simulink model "gm_sampleModel1659_sub"  (R2023a)
settings: Solver=VariableStepAuto  StartTime=0.0  StopTime=10.0  RelTol=1e-3
libraries: simulink x1
settings Model: Creator=user1  LastModifiedBy=user1
settings OptimizationCC: BlockReduction=off  ConditionallyExecuteInputs=off
settings DebuggingCC: InheritedTsInSrcMsg=none

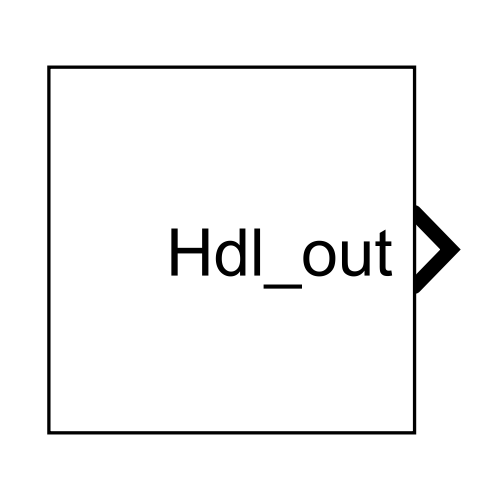
[thumbnail: Simulink's stored preview of the top-level diagram]
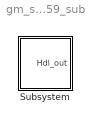
== system gm_sampleModel1659_sub ==
  Subsystem : Subsystem

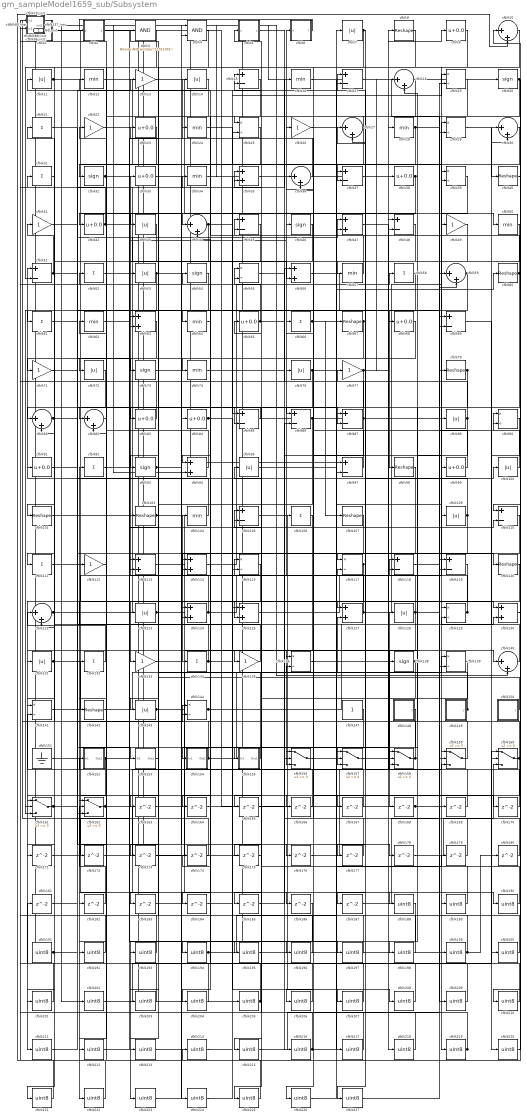
== system gm_sampleModel1659_sub/Subsystem ==
  cfblk1 : Subsystem  mask(Detect Fall Nonpositive){vinit=double(0), InputProcessing=Elements as channels (sample based), OutDataTypeStr=uint8}
      mask prompts: vinit "Simulink:masks:InitialCondition_MP"; InputProcessing "Simulink:masks:InputProcessing_MP"; OutDataTypeStr "Simulink:masks:OutputDataType_MP"
      mask help: Simulink:masks:DetectFallNonpositive_MD
      mask init:
      | InputProcessing = 'Elements as channels (sample based)';
      | OutDataTypeStr = 'uint8';
      | vinit = double(0);
      mask TypeOptions InputProcessing: Simulink:masks:ColumnsAsChannelsFrameBased | Simulink:masks:ElementsAsChannelsSampleBased
      mask TypeOptions OutDataTypeStr: Simulink:masks:uint8 | Simulink:masks:boolean
      mask Display: fprintf('U <= 0\n&  NOT\nU/z <= 0')
  cfblk{10,18,27,30,36,44,59,81..82,121,140} (11 alike) : Sum  Inputs=|++  OutDataTypeStr=uint8
  cfblk{7,11,14,43,53,72,76,89,95,100,109,123,128,131,143} (15 alike) : Abs  OutDataTypeStr=uint8  SaturateOnIntegerOverflow=off
  cfblk{8,40,60,67,79,98,101,103,107,120,142} (11 alike) : Reshape
  cfblk102_inst : Subsystem
  cfblk{12,16,24,28,34,50,57,62,64,74,104} (11 alike) : MinMax  OutDataTypeStr=uint8
  cfblk{15,17,37,45,48,51,69,85..87,97,105,110,118..119} (15 alike) : Sum  Inputs=+-  OutDataTypeStr=uint8
  cfblk{21,31,52,58,61,66,92,106,111,132,134} (11 alike) : Sum  Inputs=+  OutDataTypeStr=uint8
  cfblk108_inst : Subsystem
  cfblk{13,22,26,41,49,71,77,112,133,135} (10 alike) : Gain  OutDataTypeStr=uint8
  cfblk{35,47,56,63,94,113..114,124..125,127,130} (11 alike) : Sum  OutDataTypeStr=uint8
  cfblk{19,25,29,39,55,90,115,117,129,136,139,141,144} (13 alike) : Product  Inputs=*/  OutDataTypeStr=uint8  RndMeth=Zero  SaturateOnIntegerOverflow=on
  cfblk116_inst : Subsystem
  cfblk126_inst : Subsystem
  cfblk137_inst : Subsystem
  cfblk{20,32,46,54,73,93,138} (7 alike) : Signum
  cfblk147 : Constant  OutDataTypeStr=uint8  SampleTime=-1
  cfblk148 : Subsystem  mask(Counter Free-Running){NumBits=double(16), tsamp=double(-1)}
      mask prompts: NumBits "Simulink:masks:NumberOfBits_MP"; tsamp "Simulink:masks:SampleTime_MP"
      mask help: Simulink:masks:CounterFreeRunning_MD
  cfblk149 : Subsystem  mask(Counter Limited){uplimit=double(7), tsamp=double(-1)}
      mask prompts: uplimit "Simulink:masks:UpperLimit_MP"; tsamp "Simulink:masks:SampleTime_MP"
      mask help: Simulink:masks:CounterLimited_MD
      mask init:
      | nbits = double(8);
      | tsamp = double(-1);
      | uplimit = double(7);
  cfblk150 : Subsystem  mask(Counter Free-Running){NumBits=double(16), tsamp=double(-1)}
      mask prompts: NumBits "Simulink:masks:NumberOfBits_MP"; tsamp "Simulink:masks:SampleTime_MP"
      mask help: Simulink:masks:CounterFreeRunning_MD
  cfblk151 : Ground
  cfblk152 : Subsystem
  cfblk153 : Subsystem
  cfblk154 : Subsystem
  cfblk155 : Subsystem
  cfblk{156..162} (7 alike) : Switch  OutDataTypeStr=uint8  SaturateOnIntegerOverflow=off  InputSameDT=off
  cfblk{163..187} (25 alike) : Delay  SampleTime=1
  cfblk{188..227} (40 alike) : DataTypeConversion  OutDataTypeStr=uint8  SaturateOnIntegerOverflow=off  RndMeth=Floor
  cfblk2 : Subsystem  mask(Compare To Constant){relop=<=, const=double(3), OutDataTypeStr=uint8, ZeroCross=on}
      mask prompts: relop "Simulink:masks:Operator_MP"; const "Simulink:masks:ConstantValue_MP"; OutDataTypeStr "Simulink:masks:OutputDataType_MP"; ZeroCross "Simulink:masks:EnableZerocrossingDetection_MP"
      mask help: Simulink:masks:CompareToConstant_MD
      mask init:
      | OutDataTypeStr = 'uint8';
      | ZeroCross = 'on';
      | blkName = 'sampleModel1659_sub/Subsystem/cfblk2';
      | const = double(3);
      | const_str = '3.0';
      | const_val = double(3);
      | relop = '<=';
      | setValue = 'fixdt(0, 8)';
      | str = '<= 3';
      mask TypeOptions relop: == | ~= | < | <= | >= | >
      mask TypeOptions OutDataTypeStr: Simulink:masks:uint8 | Simulink:masks:boolean
      mask Callback ZeroCross: sl('zeroCrossEnable', gcbh);
      mask Display: disp(str)
  cfblk{9,23,33,38,42,65,68,83..84,91,99} (11 alike) : Bias  Bias=0.0  SaturateOnIntegerOverflow=off
  cfblk3 : simulink/Logic and Bit Operations/Bitwise Operator  logicop=AND  UseBitMask=on  BitMask=bin2dec('11011001')  BitMaskRealWorld=Stored Integer
      settings: LibrarySourceBlock=|
      | hdlsllib/Logic and Bit
      | Operations/Bitwise
      | Operator
  cfblk4 : Logic  AllPortsSameDT=off  OutDataTypeStr=boolean
  cfblk5 : Subsystem  mask(Compare To Constant){relop=<=, const=double(3), OutDataTypeStr=uint8, ZeroCross=on}
      mask prompts: relop "Simulink:masks:Operator_MP"; const "Simulink:masks:ConstantValue_MP"; OutDataTypeStr "Simulink:masks:OutputDataType_MP"; ZeroCross "Simulink:masks:EnableZerocrossingDetection_MP"
      mask help: Simulink:masks:CompareToConstant_MD
      mask init:
      | OutDataTypeStr = 'uint8';
      | ZeroCross = 'on';
      | blkName = 'sampleModel1659_sub/Subsystem/cfblk5';
      | const = double(3);
      | const_str = '3.0';
      | const_val = double(3);
      | relop = '<=';
      | setValue = 'fixdt(0, 8)';
      | str = '<= 3';
      mask TypeOptions relop: == | ~= | < | <= | >= | >
      mask TypeOptions OutDataTypeStr: Simulink:masks:uint8 | Simulink:masks:boolean
      mask Callback ZeroCross: sl('zeroCrossEnable', gcbh);
      mask Display: disp(str)
  cfblk6 : Subsystem  mask(Detect Rise Positive){vinit=double(0), InputProcessing=Elements as channels (sample based), OutDataTypeStr=uint8}
      mask prompts: vinit "Simulink:masks:InitialCondition_MP"; InputProcessing "Simulink:masks:InputProcessing_MP"; OutDataTypeStr "Simulink:masks:OutputDataType_MP"
      mask help: Simulink:masks:DetectRisePositive_MD
      mask init:
      | InputProcessing = 'Elements as channels (sample based)';
      | OutDataTypeStr = 'uint8';
      | vinit = double(0);
      mask TypeOptions InputProcessing: Simulink:masks:ColumnsAsChannelsFrameBased | Simulink:masks:ElementsAsChannelsSampleBased
      mask TypeOptions OutDataTypeStr: Simulink:masks:uint8 | Simulink:masks:boolean
      mask Display: fprintf('U > 0\n&  NOT\nU/z > 0')
  cfblk75_inst : Subsystem
  cfblk80_inst : Subsystem
  cfblk88_inst : Subsystem
  cfblk96_inst : Subsystem
  Hdl_out : Outport  OutDataTypeStr=uint8  SampleTime=1
  wires:
  cfblk1/1(Y) -> cfblk37/2, cfblk125/2
  cfblk10/1 -> cfblk219/1
  cfblk100/1 -> cfblk90/1
  cfblk101/1 -> cfblk33/1
  cfblk102_inst/1(out1) -> cfblk140/2
  cfblk103/1 -> cfblk190/1, cfblk157/3
  cfblk104/1 -> cfblk51/1
  cfblk105/1 -> cfblk208/1
  cfblk106/1 -> cfblk211/1
  cfblk107/1 -> cfblk134/1
  cfblk108_inst/1(out1) -> cfblk199/1
  cfblk109/1 -> cfblk27/2, cfblk215/1
  cfblk11/1 -> cfblk44/1, cfblk161/1
  cfblk110/1 -> cfblk159/1
  cfblk111/1 -> cfblk92/1
  cfblk112/1 -> cfblk22/1
  cfblk113/1 -> cfblk168/1
  cfblk114/1 -> cfblk58/1
  cfblk115/1 -> cfblk222/1
  cfblk116_inst/1(out1) -> cfblk38/1
  cfblk117/1 -> cfblk131/1, cfblk185/1, cfblk135/1
  cfblk118/1 -> cfblk169/1
  cfblk119/1 -> cfblk175/1
  cfblk12/1 -> cfblk217/1
  cfblk120/1 -> cfblk133/1
  cfblk121/1 -> cfblk47/1, cfblk129/1
  cfblk123/1 -> cfblk4/2, cfblk156/3
  cfblk124/1 -> cfblk117/2, cfblk104/1
  cfblk125/1 -> cfblk29/1
  cfblk126_inst/1(out1) -> cfblk94/2, cfblk89/1
  cfblk127/1 -> cfblk39/2, cfblk6/1(U)
  cfblk128/1 -> cfblk63/1, cfblk90/2, cfblk184/1, cfblk183/1
  cfblk129/1 -> cfblk76/1, cfblk118/1, cfblk13/1
  cfblk13/1 -> cfblk209/1
  cfblk130/1 -> cfblk214/1
  cfblk131/1 -> cfblk201/1, cfblk186/1
  cfblk132/1 -> cfblk121/1
  cfblk133/1 -> cfblk156/1
  cfblk134/1 -> cfblk91/1, cfblk207/1
  cfblk135/1 -> cfblk112/1
  cfblk136/1 -> cfblk48/2
  cfblk137_inst/1(out1) -> cfblk97/1
  cfblk138/1 -> cfblk227/1, cfblk196/1, cfblk187/1
  cfblk139/1 -> cfblk225/1
  cfblk14/1 -> cfblk182/1
  cfblk140/1 -> cfblk129/2
  cfblk141/1 -> cfblk8/1
  cfblk142/1 -> cfblk28/1
  cfblk143/1 -> cfblk69/1, cfblk127/2
  cfblk144/1 -> cfblk30/2, cfblk30/1
  cfblk147/1 -> cfblk192/1
  cfblk148/1(y) -> cfblk162/1
  cfblk149/1(y) -> cfblk36/1, cfblk103/1, cfblk77/1
  cfblk15/1 -> cfblk82/1
  cfblk150/1(y) -> cfblk53/1
  cfblk151/1 -> cfblk220/1
  cfblk152/1(Out1) -> cfblk113/1, cfblk171/1, cfblk52/1
  cfblk153/1(Out1) -> cfblk23/1
  cfblk154/1(Out1) -> cfblk59/1, cfblk31/1
  cfblk155/1(Out1) -> cfblk54/1
  cfblk156/1 -> cfblk67/1
  cfblk157/1 -> cfblk128/1
  cfblk158/1 -> cfblk17/1, cfblk116_inst/1(in1), cfblk66/1
  cfblk159/1 -> cfblk95/1
  cfblk16/1 -> cfblk157/1
  cfblk160/1 -> cfblk206/1, cfblk18/2
  cfblk161/1 -> cfblk125/1, cfblk100/1
  cfblk162/1 -> cfblk224/1, cfblk166/1
  cfblk163/1 -> cfblk29/2
  cfblk164/1 -> cfblk25/2
  cfblk165/1 -> cfblk86/2
  cfblk166/1 -> cfblk141/2
  cfblk167/1 -> cfblk15/1
  cfblk168/1 -> cfblk59/2, Hdl_out/1
  cfblk169/1 -> cfblk27/1
  cfblk17/1 -> cfblk119/1
  cfblk170/1 -> cfblk48/1
  cfblk171/1 -> cfblk63/2
  cfblk172/1 -> cfblk157/2
  cfblk173/1 -> cfblk158/2
  cfblk174/1 -> cfblk126_inst/2(in2)
  cfblk175/1 -> cfblk1/1(U)
  cfblk176/1 -> cfblk159/3
  cfblk177/1 -> cfblk156/2
  cfblk178/1 -> cfblk160/3
  cfblk179/1 -> cfblk136/2
  cfblk18/1 -> cfblk143/1
  cfblk180/1 -> cfblk159/2
  cfblk181/1 -> cfblk144/1
  cfblk182/1 -> cfblk162/2
  cfblk183/1 -> cfblk114/2
  cfblk184/1 -> cfblk130/2
  cfblk185/1 -> cfblk110/2
  cfblk186/1 -> cfblk223/1
  cfblk187/1 -> cfblk79/1
  cfblk188/1 -> cfblk193/1
  cfblk189/1 -> cfblk35/1
  cfblk19/1 -> cfblk213/1
  cfblk190/1 -> cfblk35/2
  cfblk191/1 -> cfblk47/2, cfblk34/1
  cfblk192/1 -> cfblk88_inst/1(in1)
  cfblk193/1 -> cfblk88_inst/2(in2)
  cfblk194/1 -> cfblk7/1, cfblk44/2
  cfblk195/1 -> cfblk45/1
  cfblk196/1 -> cfblk45/2
  cfblk197/1 -> cfblk3/1
  cfblk198/1 -> cfblk62/1
  cfblk199/1 -> cfblk102_inst/2(in2), cfblk180/1, cfblk12/1
  cfblk2/1(y) -> cfblk189/1
  cfblk20/1 -> cfblk94/1, cfblk210/1
  cfblk200/1 -> cfblk108_inst/1(in1)
  cfblk201/1 -> cfblk108_inst/2(in2)
  cfblk202/1 -> cfblk160/1
  cfblk203/1 -> cfblk75_inst/1(in1)
  cfblk204/1 -> cfblk75_inst/2(in2)
  cfblk205/1 -> cfblk96_inst/2(in2), cfblk181/1
  cfblk206/1 -> cfblk80_inst/1(in1)
  cfblk207/1 -> cfblk80_inst/2(in2)
  cfblk208/1 -> cfblk174/1
  cfblk209/1 -> cfblk105/1
  cfblk21/1 -> cfblk73/1
  cfblk210/1 -> cfblk105/2
  cfblk211/1 -> cfblk162/3
  cfblk212/1 -> cfblk106/1
  cfblk213/1 -> cfblk84/1
  cfblk214/1 -> cfblk19/1
  cfblk215/1 -> cfblk19/2
  cfblk216/1 -> cfblk65/1, cfblk179/1
  cfblk217/1 -> cfblk55/1
  cfblk218/1 -> cfblk55/2
  cfblk219/1 -> cfblk137_inst/1(in1), cfblk5/1(u)
  cfblk22/1 -> cfblk56/2
  cfblk220/1 -> cfblk10/1
  cfblk221/1 -> cfblk10/2
  cfblk222/1 -> cfblk126_inst/1(in1)
  cfblk223/1 -> cfblk115/1
  cfblk224/1 -> cfblk115/2
  cfblk225/1 -> cfblk152/1(In1)
  cfblk226/1 -> cfblk139/1
  cfblk227/1 -> cfblk139/2
  cfblk23/1 -> cfblk132/1
  cfblk24/1 -> cfblk39/1
  cfblk25/1 -> cfblk32/1
  cfblk26/1 -> cfblk97/2
  cfblk27/1 -> cfblk124/1, cfblk25/1
  cfblk28/1 -> cfblk87/2, cfblk130/1
  cfblk29/1 -> cfblk40/1
  cfblk3/1 -> cfblk42/1
  cfblk30/1 -> cfblk142/1
  cfblk31/1 -> cfblk61/1
  cfblk32/1 -> cfblk85/2, cfblk64/1
  cfblk33/1 -> cfblk178/1
  cfblk34/1 -> cfblk85/1
  cfblk35/1 -> cfblk188/1
  cfblk36/1 -> cfblk14/1
  cfblk37/1 -> cfblk9/1
  cfblk38/1 -> cfblk72/1, cfblk177/1
  cfblk39/1 -> cfblk49/1
  cfblk4/1 -> cfblk51/2
  cfblk40/1 -> cfblk110/1
  cfblk41/1 -> cfblk83/1
  cfblk42/1 -> cfblk124/2, cfblk102_inst/1(in1), cfblk16/1
  cfblk43/1 -> cfblk111/1
  cfblk44/1 -> cfblk82/2, cfblk69/2
  cfblk45/1 -> cfblk194/1
  cfblk46/1 -> cfblk203/1
  cfblk47/1 -> cfblk119/2
  cfblk48/1 -> cfblk93/1
  cfblk49/1 -> cfblk172/1
  cfblk5/1(y) -> cfblk50/1
  cfblk50/1 -> cfblk121/2
  cfblk51/1 -> cfblk113/2, cfblk41/1
  cfblk52/1 -> cfblk24/1
  cfblk53/1 -> cfblk161/3, cfblk155/1(In1)
  cfblk54/1 -> cfblk161/2
  cfblk55/1 -> cfblk216/1
  cfblk56/1 -> cfblk98/1
  cfblk57/1 -> cfblk11/1
  cfblk58/1 -> cfblk141/1
  cfblk59/1 -> cfblk164/1, cfblk144/2
  cfblk6/1(Y) -> cfblk2/1(u)
  cfblk60/1 -> cfblk198/1, cfblk26/1
  cfblk61/1 -> cfblk68/1
  cfblk62/1 -> cfblk197/1
  cfblk63/1 -> cfblk81/2
  cfblk64/1 -> cfblk114/1
  cfblk65/1 -> cfblk140/1, cfblk116_inst/2(in2)
  cfblk66/1 -> cfblk60/1, cfblk107/1
  cfblk67/1 -> cfblk127/1, cfblk71/1
  cfblk68/1 -> cfblk74/1
  cfblk69/1 -> cfblk200/1
  cfblk7/1 -> cfblk43/1, cfblk57/1
  cfblk71/1 -> cfblk15/2
  cfblk72/1 -> cfblk101/1
  cfblk73/1 -> cfblk167/1
  cfblk74/1 -> cfblk99/1
  cfblk75_inst/1(out1) -> cfblk202/1
  cfblk76/1 -> cfblk226/1, cfblk173/1, cfblk170/1
  cfblk77/1 -> cfblk218/1, cfblk195/1, cfblk18/1
  cfblk79/1 -> cfblk204/1, cfblk138/1, cfblk117/1
  cfblk8/1 -> cfblk86/1
  cfblk80_inst/1(out1) -> cfblk205/1
  cfblk81/1 -> cfblk176/1, cfblk153/1(In1)
  cfblk82/1 -> cfblk212/1
  cfblk83/1 -> cfblk21/1
  cfblk84/1 -> cfblk87/1, cfblk17/2, cfblk158/3
  cfblk85/1 -> cfblk81/1
  cfblk86/1 -> cfblk163/1, cfblk154/1(In1)
  cfblk87/1 -> cfblk56/1, cfblk136/1
  cfblk88_inst/1(out1) -> cfblk191/1
  cfblk89/1 -> cfblk96_inst/1(in1), cfblk4/1, cfblk158/1
  cfblk9/1 -> cfblk221/1
  cfblk90/1 -> cfblk160/2
  cfblk91/1 -> cfblk118/2
  cfblk92/1 -> cfblk46/1
  cfblk93/1 -> cfblk123/1, cfblk120/1
  cfblk94/1 -> cfblk137_inst/2(in2)
  cfblk95/1 -> cfblk109/1
  cfblk96_inst/1(out1) -> cfblk20/1
  cfblk97/1 -> cfblk36/2
  cfblk98/1 -> cfblk165/1
  cfblk99/1 -> cfblk37/1

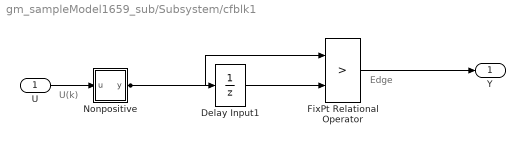
== system gm_sampleModel1659_sub/Subsystem/cfblk1 ==
  note: U(k)
  note: Edge
  U : Inport  OutDataTypeStr=uint8  SampleTime=1
  Delay Input1 : UnitDelay  Description=Store in Global RAM  DisableCoverage=on  InitialCondition=vinit  SampleTime=-1  HasFrameUpgradeWarning=on
  FixPt Relational Operator : RelationalOperator  Operator=>  OutDataTypeStr=fixdt(0, 8)  ZeroCross=off  InputSameDT=off
  Nonpositive : Subsystem  mask(Compare To Zero){relop=<=, OutDataTypeStr=boolean, ZeroCross=off}
      mask prompts: relop "Simulink:masks:Operator_MP"; OutDataTypeStr "Simulink:masks:OutputDataType_MP"; ZeroCross "Simulink:masks:EnableZerocrossingDetection_MP"
      mask help: Simulink:masks:CompareToZero_MD
      mask init:
      | OutDataTypeStr = 'boolean';
      | ZeroCross = 'off';
      | blkName = 'sampleModel1659_sub/Subsystem/cfblk1/Nonpositive';
      | relop = '<=';
      | setValue = 'boolean';
      mask TypeOptions relop: == | ~= | < | <= | >= | >
      mask TypeOptions OutDataTypeStr: Simulink:masks:uint8 | Simulink:masks:boolean
      mask Callback ZeroCross: sl('zeroCrossEnable', gcbh);
      mask Display: disp([relop,' 0'])
  Y : Outport  SampleTime=1
  wires:
  U/1 -> Nonpositive/1(u)
  Delay Input1/1 -> FixPt Relational Operator/2
  FixPt Relational Operator/1 -> Y/1
  Nonpositive/1(y) -> FixPt Relational Operator/1, Delay Input1/1

== system gm_sampleModel1659_sub/Subsystem/cfblk102_inst ==
  in1 : Inport  OutDataTypeStr=uint8  SampleTime=1
  in2 : Inport  Port=2  OutDataTypeStr=uint8  SampleTime=1
  mul_cfblk102_dotp_mulcomp : Product  Inputs=**  OutDataTypeStr=uint8  SampleTime=1
  out1 : Outport  OutDataTypeStr=uint8  SampleTime=1
  wires:
  in1/1 -> mul_cfblk102_dotp_mulcomp/1
  in2/1 -> mul_cfblk102_dotp_mulcomp/2
  mul_cfblk102_dotp_mulcomp/1 -> out1/1

== system gm_sampleModel1659_sub/Subsystem/cfblk108_inst ==
  in1 : Inport  OutDataTypeStr=uint8  SampleTime=1
  in2 : Inport  Port=2  OutDataTypeStr=uint8  SampleTime=1
  mul_cfblk108_dotp_mulcomp : Product  Inputs=**  OutDataTypeStr=uint8  SampleTime=1
  out1 : Outport  OutDataTypeStr=uint8  SampleTime=1
  wires:
  in1/1 -> mul_cfblk108_dotp_mulcomp/1
  in2/1 -> mul_cfblk108_dotp_mulcomp/2
  mul_cfblk108_dotp_mulcomp/1 -> out1/1

== system gm_sampleModel1659_sub/Subsystem/cfblk116_inst ==
  in1 : Inport  OutDataTypeStr=uint8  SampleTime=1
  in2 : Inport  Port=2  OutDataTypeStr=uint8  SampleTime=1
  mul_cfblk116_dotp_mulcomp : Product  Inputs=**  OutDataTypeStr=uint8  SampleTime=1
  out1 : Outport  OutDataTypeStr=uint8  SampleTime=1
  wires:
  in1/1 -> mul_cfblk116_dotp_mulcomp/1
  in2/1 -> mul_cfblk116_dotp_mulcomp/2
  mul_cfblk116_dotp_mulcomp/1 -> out1/1

== system gm_sampleModel1659_sub/Subsystem/cfblk126_inst ==
  in1 : Inport  OutDataTypeStr=uint8  SampleTime=1
  in2 : Inport  Port=2  OutDataTypeStr=uint8  SampleTime=1
  mul_cfblk126_dotp_mulcomp : Product  Inputs=**  OutDataTypeStr=uint8  SampleTime=1
  out1 : Outport  OutDataTypeStr=uint8  SampleTime=1
  wires:
  in1/1 -> mul_cfblk126_dotp_mulcomp/1
  in2/1 -> mul_cfblk126_dotp_mulcomp/2
  mul_cfblk126_dotp_mulcomp/1 -> out1/1

== system gm_sampleModel1659_sub/Subsystem/cfblk137_inst ==
  in1 : Inport  OutDataTypeStr=uint8  SampleTime=1
  in2 : Inport  Port=2  OutDataTypeStr=uint8  SampleTime=1
  mul_cfblk137_dotp_mulcomp : Product  Inputs=**  OutDataTypeStr=uint8  SampleTime=1
  out1 : Outport  OutDataTypeStr=uint8  SampleTime=1
  wires:
  in1/1 -> mul_cfblk137_dotp_mulcomp/1
  in2/1 -> mul_cfblk137_dotp_mulcomp/2
  mul_cfblk137_dotp_mulcomp/1 -> out1/1

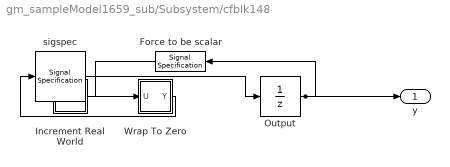
== system gm_sampleModel1659_sub/Subsystem/cfblk148 ==
  Force to be scalar : SignalSpecification  DisableCoverage=on  Dimensions=1
  Increment Real World : Subsystem  mask(Real World Value Increment){}
      mask help: Simulink:masks:RealWorldValueIncrement_MD
      mask Display: disp('V++')
  Output : UnitDelay  InitialCondition=0.0  SampleTime=tsamp  HasFrameUpgradeWarning=on
  Wrap To Zero : Subsystem  mask(Wrap To Zero){Threshold=double(65535)}
      mask prompts: Threshold "Simulink:masks:Threshold_MP"
      mask help: Simulink:masks:WrapToZero_MD
  sigspec : SignalSpecification  OutDataTypeStr=uint16  Dimensions=1
  y : Outport  SampleTime=1
  wires:
  Force to be scalar/1 -> Increment Real World/1(u)
  Increment Real World/1(y) -> Wrap To Zero/1(U)
  Output/1 -> Force to be scalar/1, y/1
  Wrap To Zero/1(Y) -> sigspec/1
  sigspec/1 -> Output/1

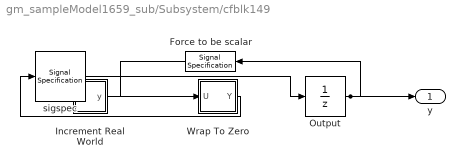
== system gm_sampleModel1659_sub/Subsystem/cfblk149 ==
  Force to be scalar : SignalSpecification  DisableCoverage=on  Dimensions=1
  Increment Real World : Subsystem  mask(Real World Value Increment){}
      mask help: Simulink:masks:RealWorldValueIncrement_MD
      mask Display: disp('V++')
  Output : UnitDelay  InitialCondition=0.0  SampleTime=tsamp  HasFrameUpgradeWarning=on
  Wrap To Zero : Subsystem  mask(Wrap To Zero){Threshold=double(7)}
      mask prompts: Threshold "Simulink:masks:Threshold_MP"
      mask help: Simulink:masks:WrapToZero_MD
  sigspec : SignalSpecification  OutDataTypeStr=uint8  Dimensions=1
  y : Outport  SampleTime=1
  wires:
  Force to be scalar/1 -> Increment Real World/1(u)
  Increment Real World/1(y) -> Wrap To Zero/1(U)
  Output/1 -> Force to be scalar/1, y/1
  Wrap To Zero/1(Y) -> sigspec/1
  sigspec/1 -> Output/1

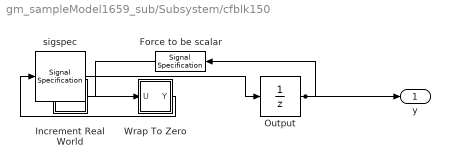
== system gm_sampleModel1659_sub/Subsystem/cfblk150 ==
  Force to be scalar : SignalSpecification  DisableCoverage=on  Dimensions=1
  Increment Real World : Subsystem  mask(Real World Value Increment){}
      mask help: Simulink:masks:RealWorldValueIncrement_MD
      mask Display: disp('V++')
  Output : UnitDelay  InitialCondition=0.0  SampleTime=tsamp  HasFrameUpgradeWarning=on
  Wrap To Zero : Subsystem  mask(Wrap To Zero){Threshold=double(65535)}
      mask prompts: Threshold "Simulink:masks:Threshold_MP"
      mask help: Simulink:masks:WrapToZero_MD
  sigspec : SignalSpecification  OutDataTypeStr=uint16  Dimensions=1
  y : Outport  SampleTime=1
  wires:
  Force to be scalar/1 -> Increment Real World/1(u)
  Increment Real World/1(y) -> Wrap To Zero/1(U)
  Output/1 -> Force to be scalar/1, y/1
  Wrap To Zero/1(Y) -> sigspec/1
  sigspec/1 -> Output/1

== system gm_sampleModel1659_sub/Subsystem/cfblk152 ==
  In1 : Inport  OutDataTypeStr=uint8  PortDimensions=1  SampleTime=1
  Out1 : Outport  SampleTime=1
  wires:
  In1/1 -> Out1/1

== system gm_sampleModel1659_sub/Subsystem/cfblk153 ==
  In1 : Inport  OutDataTypeStr=uint8  PortDimensions=1  SampleTime=1
  Out1 : Outport  SampleTime=1
  wires:
  In1/1 -> Out1/1

== system gm_sampleModel1659_sub/Subsystem/cfblk154 ==
  In1 : Inport  OutDataTypeStr=uint8  PortDimensions=1  SampleTime=1
  Out1 : Outport  SampleTime=1
  wires:
  In1/1 -> Out1/1

== system gm_sampleModel1659_sub/Subsystem/cfblk155 ==
  In1 : Inport  OutDataTypeStr=uint8  PortDimensions=1  SampleTime=1
  Out1 : Outport  SampleTime=1
  wires:
  In1/1 -> Out1/1

== system gm_sampleModel1659_sub/Subsystem/cfblk2 ==
  u : Inport  OutDataTypeStr=uint8  SampleTime=1
  Compare : RelationalOperator  Operator=<=  OutDataTypeStr=fixdt(0, 8)
  Constant : Constant  DisableCoverage=on  Value=const  OutDataTypeStr=Inherit: Inherit via back propagation  SampleTime=-1
  y : Outport  SampleTime=1
  wires:
  u/1 -> Compare/1
  Compare/1 -> y/1
  Constant/1 -> Compare/2

== system gm_sampleModel1659_sub/Subsystem/cfblk5 ==
  u : Inport  OutDataTypeStr=uint8  SampleTime=1
  Compare : RelationalOperator  Operator=<=  OutDataTypeStr=fixdt(0, 8)
  Constant : Constant  DisableCoverage=on  Value=const  OutDataTypeStr=Inherit: Inherit via back propagation  SampleTime=-1
  y : Outport  SampleTime=1
  wires:
  u/1 -> Compare/1
  Compare/1 -> y/1
  Constant/1 -> Compare/2

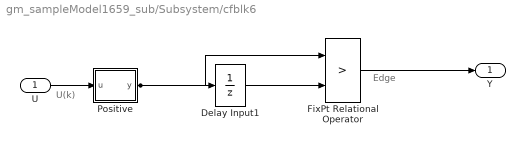
== system gm_sampleModel1659_sub/Subsystem/cfblk6 ==
  note: U(k)
  note: Edge
  U : Inport  OutDataTypeStr=uint8  SampleTime=1
  Delay Input1 : UnitDelay  Description=Store in Global RAM  DisableCoverage=on  InitialCondition=vinit  SampleTime=-1  HasFrameUpgradeWarning=on
  FixPt Relational Operator : RelationalOperator  Operator=>  OutDataTypeStr=fixdt(0, 8)  ZeroCross=off  InputSameDT=off
  Positive : Subsystem  mask(Compare To Zero){relop=>, OutDataTypeStr=boolean, ZeroCross=off}
      mask prompts: relop "Simulink:masks:Operator_MP"; OutDataTypeStr "Simulink:masks:OutputDataType_MP"; ZeroCross "Simulink:masks:EnableZerocrossingDetection_MP"
      mask help: Simulink:masks:CompareToZero_MD
      mask init:
      | OutDataTypeStr = 'boolean';
      | ZeroCross = 'off';
      | blkName = 'sampleModel1659_sub/Subsystem/cfblk6/Positive';
      | relop = '>';
      | setValue = 'boolean';
      mask TypeOptions relop: == | ~= | < | <= | >= | >
      mask TypeOptions OutDataTypeStr: Simulink:masks:uint8 | Simulink:masks:boolean
      mask Callback ZeroCross: sl('zeroCrossEnable', gcbh);
      mask Display: disp([relop,' 0'])
  Y : Outport  SampleTime=1
  wires:
  U/1 -> Positive/1(u)
  Delay Input1/1 -> FixPt Relational Operator/2
  FixPt Relational Operator/1 -> Y/1
  Positive/1(y) -> FixPt Relational Operator/1, Delay Input1/1

== system gm_sampleModel1659_sub/Subsystem/cfblk75_inst ==
  in1 : Inport  OutDataTypeStr=uint8  SampleTime=1
  in2 : Inport  Port=2  OutDataTypeStr=uint8  SampleTime=1
  mul_cfblk75_dotp_mulcomp : Product  Inputs=**  OutDataTypeStr=uint8  SampleTime=1
  out1 : Outport  OutDataTypeStr=uint8  SampleTime=1
  wires:
  in1/1 -> mul_cfblk75_dotp_mulcomp/1
  in2/1 -> mul_cfblk75_dotp_mulcomp/2
  mul_cfblk75_dotp_mulcomp/1 -> out1/1

== system gm_sampleModel1659_sub/Subsystem/cfblk80_inst ==
  in1 : Inport  OutDataTypeStr=uint8  SampleTime=1
  in2 : Inport  Port=2  OutDataTypeStr=uint8  SampleTime=1
  mul_cfblk80_dotp_mulcomp : Product  Inputs=**  OutDataTypeStr=uint8  SampleTime=1
  out1 : Outport  OutDataTypeStr=uint8  SampleTime=1
  wires:
  in1/1 -> mul_cfblk80_dotp_mulcomp/1
  in2/1 -> mul_cfblk80_dotp_mulcomp/2
  mul_cfblk80_dotp_mulcomp/1 -> out1/1

== system gm_sampleModel1659_sub/Subsystem/cfblk88_inst ==
  in1 : Inport  OutDataTypeStr=uint8  SampleTime=1
  in2 : Inport  Port=2  OutDataTypeStr=uint8  SampleTime=1
  mul_cfblk88_dotp_mulcomp : Product  Inputs=**  OutDataTypeStr=uint8  SampleTime=1
  out1 : Outport  OutDataTypeStr=uint8  SampleTime=1
  wires:
  in1/1 -> mul_cfblk88_dotp_mulcomp/1
  in2/1 -> mul_cfblk88_dotp_mulcomp/2
  mul_cfblk88_dotp_mulcomp/1 -> out1/1

== system gm_sampleModel1659_sub/Subsystem/cfblk96_inst ==
  in1 : Inport  OutDataTypeStr=uint8  SampleTime=1
  in2 : Inport  Port=2  OutDataTypeStr=uint8  SampleTime=1
  mul_cfblk96_dotp_mulcomp : Product  Inputs=**  OutDataTypeStr=uint8  SampleTime=1
  out1 : Outport  OutDataTypeStr=uint8  SampleTime=1
  wires:
  in1/1 -> mul_cfblk96_dotp_mulcomp/1
  in2/1 -> mul_cfblk96_dotp_mulcomp/2
  mul_cfblk96_dotp_mulcomp/1 -> out1/1

== system gm_sampleModel1659_sub/Subsystem/cfblk1/Nonpositive ==
  u : Inport  OutDataTypeStr=uint8  SampleTime=1
  Compare : RelationalOperator  Operator=<=  OutDataTypeStr=boolean  ZeroCross=off
  Constant : Constant  DisableCoverage=on  Value=0  OutDataTypeStr=Inherit: Inherit via back propagation  SampleTime=-1  PreserveConstantTs=on
  y : Outport  SampleTime=1
  wires:
  u/1 -> Compare/1
  Compare/1 -> y/1
  Constant/1 -> Compare/2

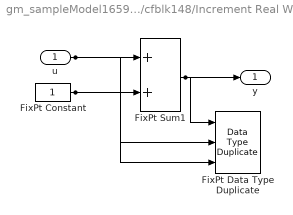
== system gm_sampleModel1659_sub/Subsystem/cfblk148/Increment Real World ==
  u : Inport  OutDataTypeStr=uint16  SampleTime=1
  FixPt Constant : Constant  DisableCoverage=on  OutDataTypeStr=Inherit: Inherit via back propagation  SampleTime=-1
  FixPt Data Type Duplicate : DataTypeDuplicate  DisableCoverage=on  NumInputPorts=3
  FixPt Sum1 : Sum  InputSameDT=on  OutDataTypeStr=Inherit: Inherit via back propagation  LockScale=on
  y : Outport  SampleTime=1
  wires:
  u/1 -> FixPt Sum1/1, FixPt Data Type Duplicate/2
  FixPt Constant/1 -> FixPt Sum1/2, FixPt Data Type Duplicate/3
  FixPt Sum1/1 -> FixPt Data Type Duplicate/1, y/1

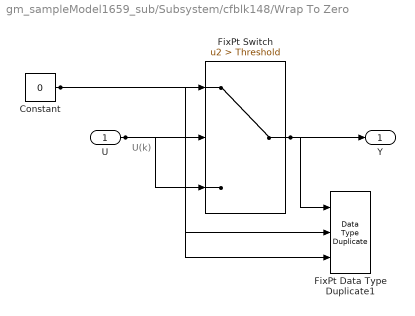
== system gm_sampleModel1659_sub/Subsystem/cfblk148/Wrap To Zero ==
  note: U(k)
  U : Inport  OutDataTypeStr=uint16  SampleTime=1
  Constant : Constant  DisableCoverage=on  Value=0  OutDataTypeStr=Inherit: Inherit via back propagation  SampleTime=-1
  FixPt Data Type Duplicate1 : DataTypeDuplicate  DisableCoverage=on  NumInputPorts=3
  FixPt Switch : Switch  Criteria=u2 > Threshold  Threshold=Threshold  OutDataTypeStr=Inherit: Inherit via back propagation  ZeroCross=off  SaturateOnIntegerOverflow=off  InputSameDT=off
  Y : Outport  SampleTime=1
  wires:
  U/1 -> FixPt Switch/3, FixPt Switch/2, FixPt Data Type Duplicate1/2
  Constant/1 -> FixPt Switch/1, FixPt Data Type Duplicate1/3
  FixPt Switch/1 -> FixPt Data Type Duplicate1/1, Y/1

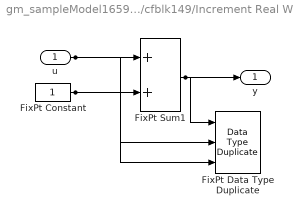
== system gm_sampleModel1659_sub/Subsystem/cfblk149/Increment Real World ==
  u : Inport  OutDataTypeStr=uint8  SampleTime=1
  FixPt Constant : Constant  DisableCoverage=on  OutDataTypeStr=Inherit: Inherit via back propagation  SampleTime=-1
  FixPt Data Type Duplicate : DataTypeDuplicate  DisableCoverage=on  NumInputPorts=3
  FixPt Sum1 : Sum  InputSameDT=on  OutDataTypeStr=Inherit: Inherit via back propagation  LockScale=on
  y : Outport  SampleTime=1
  wires:
  u/1 -> FixPt Sum1/1, FixPt Data Type Duplicate/2
  FixPt Constant/1 -> FixPt Sum1/2, FixPt Data Type Duplicate/3
  FixPt Sum1/1 -> FixPt Data Type Duplicate/1, y/1

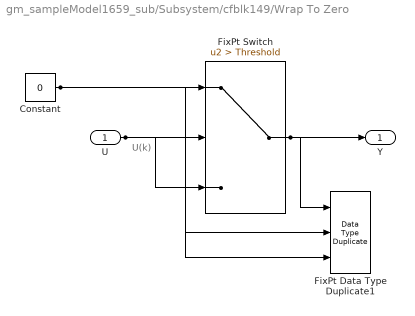
== system gm_sampleModel1659_sub/Subsystem/cfblk149/Wrap To Zero ==
  note: U(k)
  U : Inport  OutDataTypeStr=uint8  SampleTime=1
  Constant : Constant  DisableCoverage=on  Value=0  OutDataTypeStr=Inherit: Inherit via back propagation  SampleTime=-1
  FixPt Data Type Duplicate1 : DataTypeDuplicate  DisableCoverage=on  NumInputPorts=3
  FixPt Switch : Switch  Criteria=u2 > Threshold  Threshold=Threshold  OutDataTypeStr=Inherit: Inherit via back propagation  ZeroCross=off  SaturateOnIntegerOverflow=off  InputSameDT=off
  Y : Outport  SampleTime=1
  wires:
  U/1 -> FixPt Switch/3, FixPt Switch/2, FixPt Data Type Duplicate1/2
  Constant/1 -> FixPt Switch/1, FixPt Data Type Duplicate1/3
  FixPt Switch/1 -> FixPt Data Type Duplicate1/1, Y/1

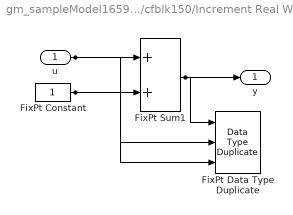
== system gm_sampleModel1659_sub/Subsystem/cfblk150/Increment Real World ==
  u : Inport  OutDataTypeStr=uint16  SampleTime=1
  FixPt Constant : Constant  DisableCoverage=on  OutDataTypeStr=Inherit: Inherit via back propagation  SampleTime=-1
  FixPt Data Type Duplicate : DataTypeDuplicate  DisableCoverage=on  NumInputPorts=3
  FixPt Sum1 : Sum  InputSameDT=on  OutDataTypeStr=Inherit: Inherit via back propagation  LockScale=on
  y : Outport  SampleTime=1
  wires:
  u/1 -> FixPt Sum1/1, FixPt Data Type Duplicate/2
  FixPt Constant/1 -> FixPt Sum1/2, FixPt Data Type Duplicate/3
  FixPt Sum1/1 -> FixPt Data Type Duplicate/1, y/1

== system gm_sampleModel1659_sub/Subsystem/cfblk150/Wrap To Zero ==
  note: U(k)
  U : Inport  OutDataTypeStr=uint16  SampleTime=1
  Constant : Constant  DisableCoverage=on  Value=0  OutDataTypeStr=Inherit: Inherit via back propagation  SampleTime=-1
  FixPt Data Type Duplicate1 : DataTypeDuplicate  DisableCoverage=on  NumInputPorts=3
  FixPt Switch : Switch  Criteria=u2 > Threshold  Threshold=Threshold  OutDataTypeStr=Inherit: Inherit via back propagation  ZeroCross=off  SaturateOnIntegerOverflow=off  InputSameDT=off
  Y : Outport  SampleTime=1
  wires:
  U/1 -> FixPt Switch/3, FixPt Switch/2, FixPt Data Type Duplicate1/2
  Constant/1 -> FixPt Switch/1, FixPt Data Type Duplicate1/3
  FixPt Switch/1 -> FixPt Data Type Duplicate1/1, Y/1

== system gm_sampleModel1659_sub/Subsystem/cfblk6/Positive ==
  u : Inport  OutDataTypeStr=uint8  SampleTime=1
  Compare : RelationalOperator  Operator=>  OutDataTypeStr=boolean  ZeroCross=off
  Constant : Constant  DisableCoverage=on  Value=0  OutDataTypeStr=Inherit: Inherit via back propagation  SampleTime=-1  PreserveConstantTs=on
  y : Outport  SampleTime=1
  wires:
  u/1 -> Compare/1
  Compare/1 -> y/1
  Constant/1 -> Compare/2
